simulink model "EnvT"  (R2016b)
settings: Solver=VariableStepAuto  StartTime=0.0  StopTime=10.0  RelTol=1e-3
settings Model: Creator=jiakui  LastModifiedBy=jiakui

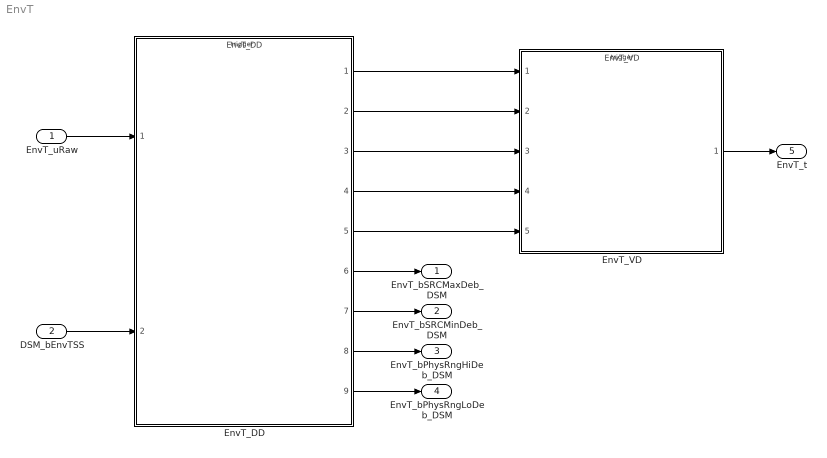
== system EnvT ==
  EnvT_uRaw : Inport  Tag=mv  Description=Sensor signal raw voltage  OutMin=0  OutMax=5000  OutDataTypeStr=Ad_mv
  DSM_bEnvTSS : Inport  Description=state of FId_EnvTSS  Port=2  OutMin=0  OutMax=1  OutDataTypeStr=boolean
  EnvT_DD : ModelReference  ModelNameDialog=EnvT_DD  SimulationMode=Normal  ModelReferenceVersion=1.12  TriggerPortName=function  TriggerPortTriggerType=function-call  TriggerPortStatesWhenEnabling=held
  EnvT_VD : ModelReference  ModelNameDialog=EnvT_VD  SimulationMode=Normal  ModelReferenceVersion=1.9  TriggerPortName=function  TriggerPortTriggerType=function-call  TriggerPortStatesWhenEnabling=held
  EnvT_bSRCMaxDeb_DSM : Outport  Description=SRC-Max error of Environment temperature sensor  OutMin=0  OutMax=1  OutDataTypeStr=boolean
  EnvT_bSRCMinDeb_DSM : Outport  Description=SRC-Min error of Environment temperature sensor  Port=2  OutMin=0  OutMax=1  OutDataTypeStr=boolean
  EnvT_bPhysRngHiDeb_DSM : Outport  Description=Physical-High of Environment temperature sensor  Port=3  OutMin=0  OutMax=1  OutDataTypeStr=boolean
  EnvT_bPhysRngLoDeb_DSM : Outport  Description=Physical-Low of Environment temperature sensor  Port=4  OutMin=0  OutMax=1  OutDataTypeStr=boolean
  EnvT_t : Outport  Tag=deg  Description=Environmental temperature  Port=5  OutMin=-200  OutMax=200  OutDataTypeStr=Temp_deg
  wires:
  EnvT_uRaw/1 -> EnvT_DD/1
  DSM_bEnvTSS/1 -> EnvT_DD/2
  EnvT_DD/1 -> EnvT_VD/1
  EnvT_DD/2 -> EnvT_VD/2
  EnvT_DD/3 -> EnvT_VD/3
  EnvT_DD/4 -> EnvT_VD/4
  EnvT_DD/5 -> EnvT_VD/5
  EnvT_DD/6 -> EnvT_bSRCMaxDeb_DSM/1
  EnvT_DD/7 -> EnvT_bSRCMinDeb_DSM/1
  EnvT_DD/8 -> EnvT_bPhysRngHiDeb_DSM/1
  EnvT_DD/9 -> EnvT_bPhysRngLoDeb_DSM/1
  EnvT_VD/1 -> EnvT_t/1
